simulink library "dspbuff2"  (Simulink 4.00)
libraries: dspbuff2 x3
settings Model: RequirementInfo=9  Creator=szlotkin  LastModifiedBy=rajbabu

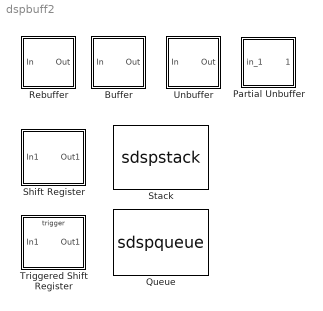
== system dspbuff2 ==
  Buffer : Subsystem  mask(Buffer){N=32, V=0, ic=0}
      mask prompts: N "Buffer size:"; V "Buffer overlap:"; ic "Initial conditions:"
      mask help: Convert scalar samples to a frame output at a lower sample rate.
      mask init:
      | [x,y] = dspblkbuff('icon');
      settings: RTWFcnNameOpts=Auto  RTWFileNameOpts=Auto
      mask Help: web(dspbhelp);
      mask Display: plot(x,y)
  Partial Unbuffer : Subsystem  mask(Partial Unbuffer){N=32, N1=13, N2=20, ic=0, num_chans=1}
      mask prompts: N "Buffer size:"; N1 "First output index:"; N2 "Last output index:"; ic "Initial conditions:"; num_chans "Number of channels"
      mask help: Convert selected portion of a frame to scalar samples output at a higher sample rate.
      mask init:
      | elements=repmat(0:N:(num_chans-1)*N,N2-N1+1,1);
      | elements=elements(:)';
      | elements=elements + repmat(N1:N2,1,num_chans);
      settings: RTWFcnNameOpts=Auto  RTWFileNameOpts=Auto
      mask Help: web(dspbhelp);
      mask Display: plot(0,0,100,100,[62 68 68 72 68 68],[24 24 26 24 22 24],[36 36 56 49 56 49],[32 24 24 16 24 32],[20 52 52 20 20],[88 88 36 36 88],[28 44],[80 80],[28 44],[72 72],[28 44],[64 64],[28 44],[56 56],[28 44],[48 48],[72 76 76 80 76 76],[24 24 26 24 22 24],[80 84 84 88 84 84],[24 24 26 24 22 24],[],[],[],[],[88 88 92],[24 24 24])
  Queue : S-Function  FunctionName=sdspqueue  Parameters=trigger,depth,overflow,pes,eso,fso,nso,clr,clrOutport  PortCounts=[]  mask(Queue){depth=8, trigger=Rising edge, overflow=Dynamic reallocation, pes=Warning, eso=off, fso=off, nso=off, clr=off, clrOutport=off}
      mask prompts: depth "Register size:"; trigger "Trigger type:"; overflow "Push onto full register:"; pes "Pop empty register:"; eso "Empty register output"; fso "Full register output"; nso "Output number of register entries"; clr "Clear input"; clrOutport "Clear output port on reset"
      mask help: Implements a queue, or "First In, First Out" (FIFO) register.
      mask init:
      | [si,so] = dspblkstack('icon', clr,eso,fso,nso);
      mask Help: web(dspbhelp);
      mask StyleString: edit,popup(Rising edge|Falling edge|Either edge),popup(Dynamic reallocation|Ignore|Warning|Error),popup(Ignore|Warning|Error),checkbox,checkbox,checkbox,checkbox,checkbox
      mask Display:
      | disp('Queue');
      | 
      | port_label('input',si(1).port, si(1).txt);
      | port_label('input',si(2).port, si(2).txt);
      | port_label('input',si(3).port, si(3).txt);
      | port_label('input',si(4).port, si(4).txt);
      | 
      | port_label('output',so(1).port, so(1).txt);
      | port_label('output',so(2).port, so(2).txt);
      | port_label('output',so(3).port, so(3).txt);
      | port_label('output',so(4).port, so(4).txt);
  Rebuffer : Subsystem  mask(Rebuffer){Specify_Out_Size=on, N=64, V=0, ic=0, frame=off, num_chans=1}
      mask prompts: Specify_Out_Size "Specify output buffer size"; N "Output buffer size (per channel):"; V "Buffer overlap:"; ic "Initial conditions:"; frame "Frame-based inputs"; num_chans "Number of channels:"
      mask help:
      | Convert a frame to a smaller or larger size with optional overlap.
      | For calculation of sample delay, see the rebuffer_delay function.
      settings: RTWFcnNameOpts=Auto  RTWFileNameOpts=Auto
      mask Help: web(dspbhelp);
      mask CallbackString: dspblkrebuff||||dspblkrebuff|
      mask Display: disp('Rebuffer')
  Shift Register : Subsystem  mask(Shift Register){siz=64, ic=0}
      mask prompts: siz "Register size:"; ic "Initial condition:"
      mask help: Shift contents of memory register and store input sample into start of register. Vector inputs are stored into independent shift registers.
      settings: RTWFcnNameOpts=Auto  RTWFileNameOpts=Auto
      mask Help: web(dspbhelp);
      mask Display: disp('Shift\nRegister');
  Stack : S-Function  FunctionName=sdspstack  Parameters=trigger,depth,overflow,pes,eso,fso,nso,clr,clrOutport  PortCounts=[]  mask(Stack){depth=8, trigger=Rising edge, overflow=Dynamic reallocation, pes=Warning, eso=off, fso=off, nso=off, clr=off, clrOutport=off}
      mask prompts: depth "Stack depth:"; trigger "Trigger type:"; overflow "Push full stack:"; pes "Pop empty stack:"; eso "Empty stack output"; fso "Full stack output"; nso "Output number of stack entries"; clr "Clear input"; clrOutport "Clear output port on reset"
      mask help: Implements a stack, or "Last In, First Out" (LIFO) register.
      mask init:
      | [si,so] = dspblkstack('icon', clr,eso,fso,nso);
      mask Help: web(dspbhelp);
      mask StyleString: edit,popup(Rising edge|Falling edge|Either edge),popup(Dynamic reallocation|Ignore|Warning|Error),popup(Ignore|Warning|Error),checkbox,checkbox,checkbox,checkbox,checkbox
      mask Display:
      | disp('Stack');
      | 
      | port_label('input',si(1).port, si(1).txt);
      | port_label('input',si(2).port, si(2).txt);
      | port_label('input',si(3).port, si(3).txt);
      | port_label('input',si(4).port, si(4).txt);
      | 
      | port_label('output',so(1).port, so(1).txt);
      | port_label('output',so(2).port, so(2).txt);
      | port_label('output',so(3).port, so(3).txt);
      | port_label('output',so(4).port, so(4).txt);
  Triggered Shift Register : Subsystem  TreatAsAtomicUnit=on  mask(Triggered Shift Register){trig=Rising edge, siz=64, ic=0}
      mask prompts: trig "Trigger type:"; siz "Register size:"; ic "Initial condition:"
      mask help: Shift contents of memory register and store input sample into start of register when trigger event occurs. Vector inputs are stored into independent shift registers.
      mask init:
      | switch trig
      | case 1, s='rising';
      | case 2, s='falling';
      | case 3, s='either';
      | end
      | set_param([gcb '/Trigger'],'triggertype',s);
      settings: RTWFcnNameOpts=Auto  RTWFileNameOpts=Auto
      mask Help: web(dspbhelp);
      mask StyleString: popup(Rising edge|Falling edge|Either edge),edit,edit
      mask Display: disp('Shift\nRegister');
  Unbuffer : Subsystem  mask(Unbuffer){ic=0, num_chans=1}
      mask prompts: ic "Initial conditions:"; num_chans "Number of channels:"
      mask help: Convert a frame to scalar samples output at a higher sample rate.
      settings: RTWFcnNameOpts=Auto  RTWFileNameOpts=Auto
      mask Help: web(dspbhelp);
      mask Display: plot(0,0,100,100,[62 68 68 72 68 68],[24 24 26 24 22 24],[36 36 56 49 56 49],[32 24 24 16 24 32],[20 52 52 20 20],[88 88 36 36 88],[28 44],[80 80],[28 44],[72 72],[28 44],[64 64],[28 44],[56 56],[28 44],[48 48],[72 76 76 80 76 76],[24 24 26 24 22 24],[80 84 84 88 84 84],[24 24 26 24 22 24],[],[],[],[],[88 88 92],[24 24 24])

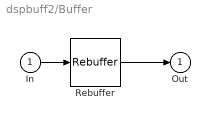
== system dspbuff2/Buffer ==
  In : Inport  Port=1
  Rebuffer : dspbuff2/Rebuffer  Specify_Out_Size=on  N=N  V=V  ic=ic  frame=off  num_chans=1
  Out : Outport  Port=1  InitialOutput=0
  wires:
  In/1 -> Rebuffer/1
  Rebuffer/1 -> Out/1

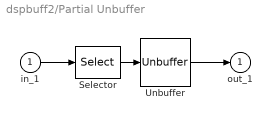
== system dspbuff2/Partial Unbuffer ==
  in_1 : Inport  Port=1
  Selector : Selector  InputType=Vector  ElementSrc=Internal  Elements=elements  RowSrc=Internal  Rows=1  ColumnSrc=Internal  Columns=1  InputPortWidth=N*num_chans
  Unbuffer : dspbuff2/Unbuffer  ic=ic  num_chans=num_chans
  out_1 : Outport  Port=1  InitialOutput=0
  wires:
  in_1/1 -> Selector/1
  Selector/1 -> Unbuffer/1
  Unbuffer/1 -> out_1/1

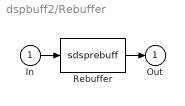
== system dspbuff2/Rebuffer ==
  In : Inport  Port=1
  Rebuffer : S-Function  FunctionName=sdsprebuff  Parameters=Specify_Out_Size,N,V,ic,frame,num_chans  PortCounts=[]
  Out : Outport  Port=1  InitialOutput=0
  wires:
  In/1 -> Rebuffer/1
  Rebuffer/1 -> Out/1

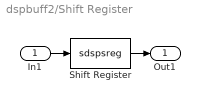
== system dspbuff2/Shift Register ==
  In1 : Inport  Port=1
  Shift Register : S-Function  FunctionName=sdspsreg  Parameters=siz,ic  PortCounts=[]
  Out1 : Outport  Port=1  InitialOutput=0
  wires:
  In1/1 -> Shift Register/1
  Shift Register/1 -> Out1/1

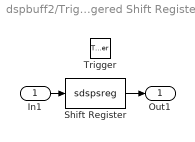
== system dspbuff2/Triggered Shift Register ==
  In1 : Inport  Port=1
  Trigger : TriggerPort  TriggerType=rising  OutputDataType=auto
  Shift Register : S-Function  FunctionName=sdspsreg  Parameters=siz,ic  PortCounts=[]
  Out1 : Outport  Port=1  InitialOutput=ic
  wires:
  Shift Register/1 -> Out1/1
  In1/1 -> Shift Register/1

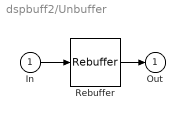
== system dspbuff2/Unbuffer ==
  In : Inport  Port=1
  Rebuffer : dspbuff2/Rebuffer  Specify_Out_Size=on  N=1  V=0  ic=ic  frame=on  num_chans=num_chans
  Out : Outport  Port=1  InitialOutput=0
  wires:
  Rebuffer/1 -> Out/1
  In/1 -> Rebuffer/1
